simulink model "VSI_sw"  (R2019a)
settings: Solver=ode23t  StartTime=0  StopTime=0.2  MaxStep=2e-6  RelTol=1e-4  AbsTol=1e-5  EnableMultiTasking=on
values from neighbouring files (symbols this model uses):
  C = 22e-6    (= 2.2e-05)    [VSI_parameters_init.m]
  Ddref = 0.355    [VSI_parameters_init.m]
  Dqref = 0.11    [VSI_parameters_init.m]
  DT = 1e-6    (= 1e-06)    [VSI_parameters_init.m]
  fsw = 20e+3    (= 20000)    [VSI_parameters_init.m]
  Idref = 3*sqrt(3)    [VSI_parameters_init.m]
  Iqref = 0    [VSI_parameters_init.m]
  kii = 2*pi*fi*(RL)/Vdcref    (= 1.0471975512)    [VSI_parameters_init.m]
  kiv = 2*pi*fv/R    (= 41.8879020479)    [VSI_parameters_init.m]
  kpi = 2*pi*fi*L/Vdcref    (= 0.0251327412287)    [VSI_parameters_init.m]
  kpv = 2*pi*fv*C    (= 0.0138230076758)    [VSI_parameters_init.m]
  L = 1.2e-3    (= 0.0012)    [VSI_parameters_init.m]
  R = 15    [VSI_parameters_init.m]
  RL = 50e-3    (= 0.05)    [VSI_parameters_init.m]
  Vdc = 300    [VSI_parameters_init.m]
  Vdcref = 300    [VSI_parameters_init.m]
  Vdref = Vsdq(1)    [VSI_parameters_init.m]
  Vfd = 0.7    [VSI_parameters_init.m]
  Vfs = 1.2    [VSI_parameters_init.m]
  Vqref = Vsdq(2)    [VSI_parameters_init.m]
  w = 2*pi*f    (= 2513.27412287)    [VSI_parameters_init.m]
libraries: powerlib x20, simulink x2
settings Model: Creator=marko  LastModifiedBy=Dominion
settings SolverCC: AutoScaleAbsTol=off  MaxConsecutiveMinStep=10
settings DataIOCC: SaveFinalState=on  SaveFormat=Array  SignalLoggingSaveFormat=ModelDataLogs  ReturnWorkspaceOutputs=off
settings OptimizationCC: ExpressionDepthLimit=2147483647  LifeSpan=inf
settings DebuggingCC: UnderspecifiedInitializationDetection=Classic  MergeDetectMultiDrivingBlocksExec=none  SolverPrmCheckMsg=warning  FcnCallInpInsideContextMsg=warning  StateNameClashWarn=warning  SFUnexpectedBacktrackingDiag=warning  SFNoUnconditionalDefaultTransitionDiag=warning  SFExecutionAtInitializationDiag=none  ArithmeticOperatorsInVariantConditions=warning
settings HardwareCC: ProdBitPerPointer=32  ProdBitPerSizeT=32  ProdBitPerPtrDiffT=32  ProdLargestAtomicFloat=None  ProdIntDivRoundTo=Undefined  ProdEndianess=Unspecified  ProdWordSize=32  ProdHWDeviceType=32-bit Generic
settings ModelReferenceCC: PropagateSignalLabelsOutOfModel=off
settings SFSimCC: SimUseLocalCustomCode=off
settings RTWCC: RTWUseLocalCustomCode=off
settings CodeAppCC: StateflowObjectComments=on
settings GRTTargetCC: TargetLangStandard=C89/C90 (ANSI)  GeneratePreprocessorConditionals=Disable all  CombineOutputUpdateFcns=off  GRTInterface=on
settings ConfigComp: CovMetricSettings=dw  CovHtmlReporting=on  CovSaveCumulativeToWorkspaceVar=on  CovSaveSingleToWorkspaceVar=on  CovExternalEMLEnable=off

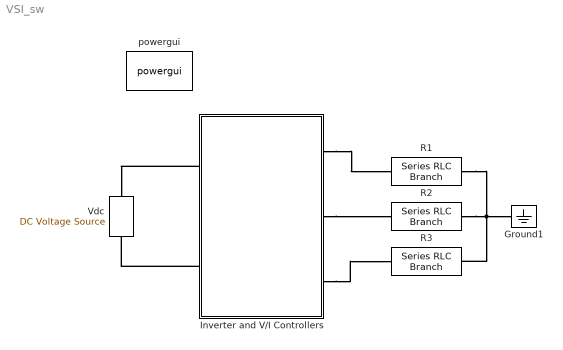
== system VSI_sw ==
  Ground1 : powerlib/Elements/Ground  LConnTagsString=a
      settings: SourceProductName=Simscape Electrical
  Inverter and V/I Controllers : Subsystem
  R1 : powerlib/Elements/Series RLC Branch  LConnTagsString=__new0  RConnTagsString=__new0  BranchType=RL  Resistance=R  Inductance=0.1*L  SetiL0=off  InitialCurrent=0  Capacitance=1e-6  Setx0=off  InitialVoltage=0  Measurements=None
      settings: SourceProductName=Simscape Electrical
  R2 : powerlib/Elements/Series RLC Branch  LConnTagsString=__new0  RConnTagsString=__new0  BranchType=RL  Resistance=R  Inductance=0.1*L  SetiL0=off  InitialCurrent=0  Capacitance=1e-6  Setx0=off  InitialVoltage=0  Measurements=None
      settings: SourceProductName=Simscape Electrical
  R3 : powerlib/Elements/Series RLC Branch  LConnTagsString=__new0  RConnTagsString=__new0  BranchType=RL  Resistance=R  Inductance=0.1*L  SetiL0=off  InitialCurrent=0  Capacitance=1e-6  Setx0=off  InitialVoltage=0  Measurements=None
      settings: SourceProductName=Simscape Electrical
  Vdc : powerlib/Electrical Sources/DC Voltage Source  Amplitude=Vdc  Measurements=None
      settings: SourceProductName=Simscape Electrical
  powergui : powerlib/powergui  Priority=1  SimulationMode=Continuous  SampleTime=50e-6  frequency=60  Iterations=50  frequencyindice=0  Pbase=100e6  ErrMax=1e-4  UnitsV=kV  UnitsW=MW  buscounter=0  FunctionMessages=off  echomessages=off  EnableUseOfTLC=off  CurrentSourceSwitches=off  DisableSnubberDevices=off  DisableRonSwitches=off  DisableVfSwitches=off  DisplayEquations=off  AutomaticDiscreteSolvers=off  SolverType=Tustin/Backward Euler (TBE)  Interpol=off  ExternalGateDelay=off  methode=off  Ts=0  x0status=blocks  SPID=on  SwTol=0  HookPort=off  NonlinearTolerance=0  nMaxIteration=15  ContinueOnMaxIteration=off  RestoreLinks=warning  ResistiveCurrentMeasurement=off  Frange=[0:2:500]  Ylog=off  Xlog=on  ShowGrid=off  save=off  variable=ZData  structure=0  ZoomFFT=on  StartTime=0.0  cycles=1  DisplayStyle=1  fundamental=60  FreqAxis=off  MaxFrequency=1000  frequencyindicesteady=400  RmsSteady=1  display=off
      settings: SourceProductName=Simscape Electrical
  connections:
  Inverter and V/I Controllers/LConn1 -- Vdc/RConn1
  Inverter and V/I Controllers/LConn2 -- Vdc/LConn1
  R1/RConn1 -- R3/RConn1 -- Ground1/LConn1 -- R2/RConn1
  Inverter and V/I Controllers/RConn1 -- R1/LConn1
  Inverter and V/I Controllers/RConn2 -- R2/LConn1
  Inverter and V/I Controllers/RConn3 -- R3/LConn1

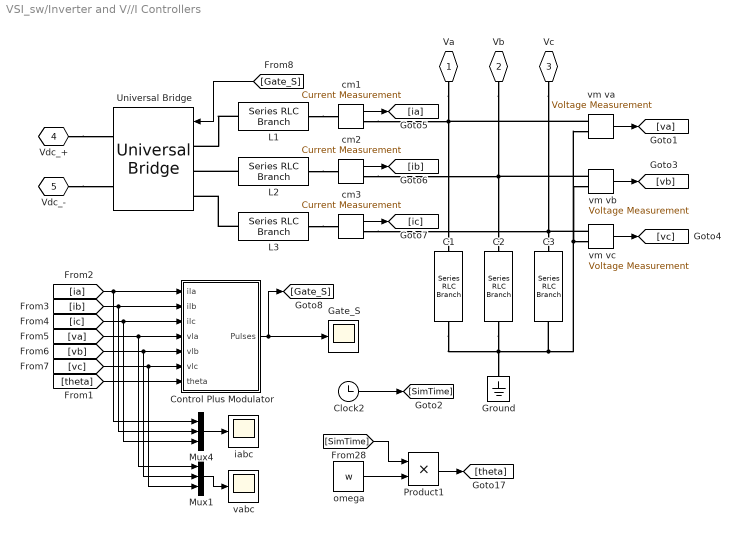
== system VSI_sw/Inverter and V//I Controllers ==
  C1 : powerlib/Elements/Series RLC Branch  LConnTagsString=__new0  RConnTagsString=__new0  BranchType=C  Resistance=1  Inductance=1e-3  SetiL0=off  InitialCurrent=0  Capacitance=C  Setx0=off  InitialVoltage=0  Measurements=None
      settings: SourceProductName=Simscape Electrical
  C2 : powerlib/Elements/Series RLC Branch  LConnTagsString=__new0  RConnTagsString=__new0  BranchType=C  Resistance=1  Inductance=1e-3  SetiL0=off  InitialCurrent=0  Capacitance=C  Setx0=off  InitialVoltage=0  Measurements=None
      settings: SourceProductName=Simscape Electrical
  C3 : powerlib/Elements/Series RLC Branch  LConnTagsString=__new0  RConnTagsString=__new0  BranchType=C  Resistance=1  Inductance=1e-3  SetiL0=off  InitialCurrent=0  Capacitance=C  Setx0=off  InitialVoltage=0  Measurements=None
      settings: SourceProductName=Simscape Electrical
  Clock2 : Clock
  Control Plus Modulator : Subsystem
  Gate_S : Scope
  Ground : powerlib/Elements/Ground  LConnTagsString=a
      settings: SourceProductName=Simscape Electrical
  L1 : powerlib/Elements/Series RLC Branch  LConnTagsString=__new0  RConnTagsString=__new0  BranchType=RL  Resistance=RL  Inductance=L  SetiL0=off  InitialCurrent=0  Capacitance=1e-6  Setx0=off  InitialVoltage=0  Measurements=None
      settings: SourceProductName=Simscape Electrical
  L2 : powerlib/Elements/Series RLC Branch  LConnTagsString=__new0  RConnTagsString=__new0  BranchType=RL  Resistance=RL  Inductance=L  SetiL0=off  InitialCurrent=0  Capacitance=1e-6  Setx0=off  InitialVoltage=0  Measurements=None
      settings: SourceProductName=Simscape Electrical
  L3 : powerlib/Elements/Series RLC Branch  LConnTagsString=__new0  RConnTagsString=__new0  BranchType=RL  Resistance=RL  Inductance=L  SetiL0=off  InitialCurrent=0  Capacitance=1e-6  Setx0=off  InitialVoltage=0  Measurements=None
      settings: SourceProductName=Simscape Electrical
  Mux1 : Mux  Inputs=3
  Mux4 : Mux  Inputs=3
  Product1 : Product  RndMeth=Zero
  Universal Bridge : powerlib/Power Electronics/Universal Bridge  Arms=3  SnubberResistance=inf  SnubberCapacitance=inf  Device=IGBT / Diodes  Ron=Rsd  Lon=0  ForwardVoltages=[Vfs Vfd]  ForwardVoltage=0  GTOparameters=[ 10e-6 , 20e-6 ]  IGBTparameters=[ 0, 0 ]  Measurements=None  Measurements_2=None  converterType=Rectifier
      settings: SourceProductName=Simscape Electrical
  cm1 : powerlib/Measurements/Current Measurement  PhasorSimulation=off  OutputType=Complex  PSBequivalent=0
      settings: SourceProductName=Simscape Electrical
  cm2 : powerlib/Measurements/Current Measurement  PhasorSimulation=off  OutputType=Complex  PSBequivalent=0
      settings: SourceProductName=Simscape Electrical
  cm3 : powerlib/Measurements/Current Measurement  PhasorSimulation=off  OutputType=Complex  PSBequivalent=0
      settings: SourceProductName=Simscape Electrical
  iabc : Scope
  omega : Constant  Value=w
  vabc : Scope
  vm va : powerlib/Measurements/Voltage Measurement  PhasorSimulation=off  OutputType=Complex  PSBequivalent=0
      settings: SourceProductName=Simscape Electrical
  vm vb : powerlib/Measurements/Voltage Measurement  PhasorSimulation=off  OutputType=Complex  PSBequivalent=0
      settings: SourceProductName=Simscape Electrical
  vm vc : powerlib/Measurements/Voltage Measurement  PhasorSimulation=off  OutputType=Complex  PSBequivalent=0
      settings: SourceProductName=Simscape Electrical
  Va : PMIOPort  Tag=PMCPort  Side=Right
  Vb : PMIOPort  Tag=PMCPort  Port=2  Side=Right
  Vc : PMIOPort  Tag=PMCPort  Port=3  Side=Right
  Vdc_+ : PMIOPort  Tag=PMCPort  Port=4  Side=Left
  Vdc_- : PMIOPort  Tag=PMCPort  Port=5  Side=Left
  wires:
  omega/1 -> Product1/2
  [SimTime] -> Product1/1
  Clock2/1 -> [SimTime]
  Product1/1 -> [theta]
  [theta] -> Control Plus Modulator/7(theta)
  Control Plus Modulator/1(Pulses) -> Gate_S/1, [Gate_S]
  Mux4/1 -> iabc/1
  vm va/1 -> [va]
  vm vb/1 -> [vb]
  vm vc/1 -> [vc]
  cm1/1 -> [ia]
  cm2/1 -> [ib]
  cm3/1 -> [ic]
  [ia] -> Control Plus Modulator/1(ila), Mux4/1
  [ib] -> Control Plus Modulator/2(ilb), Mux4/2
  [ic] -> Control Plus Modulator/3(ilc), Mux4/3
  [va] -> Control Plus Modulator/4(vla), Mux1/1
  [vb] -> Control Plus Modulator/5(vlb), Mux1/2
  [vc] -> Control Plus Modulator/6(vlc), Mux1/3
  Mux1/1 -> vabc/1
  [Gate_S] -> Universal Bridge/1
  connections:
  Va/RConn1 -- cm1/RConn1 -- C1/LConn1 -- vm va/LConn1
  C1/RConn1 -- C2/RConn1 -- Ground/LConn1 -- C3/RConn1 -- vm va/LConn2 -- vm vb/LConn2 -- vm vc/LConn2
  Vb/RConn1 -- cm2/RConn1 -- C2/LConn1 -- vm vb/LConn1
  Vc/RConn1 -- cm3/RConn1 -- C3/LConn1 -- vm vc/LConn1
  L1/LConn1 -- Universal Bridge/LConn1
  L1/RConn1 -- cm1/LConn1
  L2/LConn1 -- Universal Bridge/LConn2
  L2/RConn1 -- cm2/LConn1
  L3/LConn1 -- Universal Bridge/LConn3
  L3/RConn1 -- cm3/LConn1
  Vdc_+/RConn1 -- Universal Bridge/RConn1
  Vdc_-/RConn1 -- Universal Bridge/RConn2

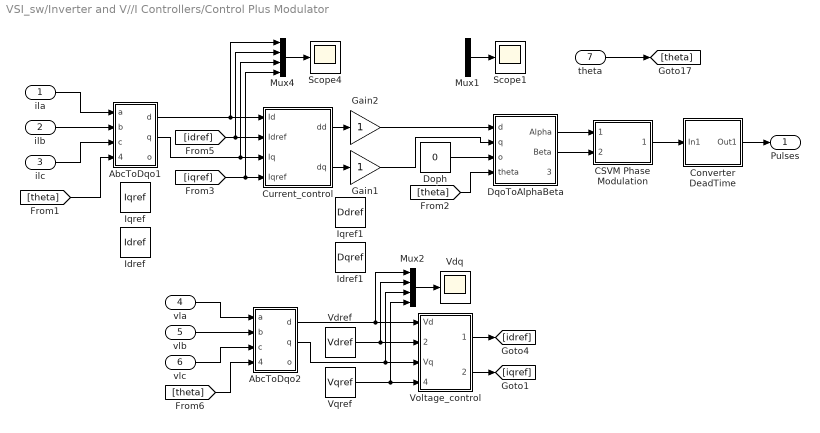
== system VSI_sw/Inverter and V//I Controllers/Control Plus Modulator ==
  ila : Inport
  ilb : Inport  Port=2
  ilc : Inport  Port=3
  vla : Inport  Port=4
  vlb : Inport  Port=5
  vlc : Inport  Port=6
  theta : Inport  Port=7
  AbcToDqo1 : Subsystem
  AbcToDqo2 : Subsystem
  CSVM Phase Modulation : Subsystem
  Converter DeadTime : Subsystem
  Current_control : Subsystem
  Doph : Constant  Value=0
  DqoToAlphaBeta : Subsystem
  Gain1 : Gain
  Gain2 : Gain
  Idref : Constant  Value=Idref
  Idref1 : Constant  Value=Dqref
  Iqref : Constant  Value=Iqref
  Iqref1 : Constant  Value=Ddref
  Mux1 : Mux  Inputs=2
  Mux2 : Mux
  Mux4 : Mux
  Scope1 : Scope
  Scope4 : Scope
  Vdq : Scope
  Vdref : Constant  Value=Vdref
  Voltage_control : Subsystem
  Vqref : Constant  Value=Vqref
  Pulses : Outport
  wires:
  AbcToDqo1/1(d) -> Current_control/1(Id), Mux4/1
  AbcToDqo1/2(q) -> Current_control/3(Iq), Mux4/3
  Current_control/1(dd) -> Gain2/1
  Current_control/2(dq) -> Gain1/1
  Mux4/1 -> Scope4/1
  ila/1 -> AbcToDqo1/1(a)
  ilb/1 -> AbcToDqo1/2(b)
  ilc/1 -> AbcToDqo1/3(c)
  theta/1 -> [theta]
  [theta] -> AbcToDqo1/4(theta)
  Mux1/1 -> Scope1/1
  DqoToAlphaBeta/1(Alpha) -> CSVM Phase Modulation/1(Dalpha)
  DqoToAlphaBeta/2(Beta) -> CSVM Phase Modulation/2(Dbeta)
  Doph/1 -> DqoToAlphaBeta/3(o)
  CSVM Phase Modulation/1(Pulses) -> Converter DeadTime/1(In1)
  [theta] -> DqoToAlphaBeta/4(theta)
  Converter DeadTime/1(Out1) -> Pulses/1
  Vqref/1 -> Voltage_control/4(Vqref), Mux2/4
  Vdref/1 -> Voltage_control/2(Vdref), Mux2/2
  AbcToDqo2/1(d) -> Voltage_control/1(Vd), Mux2/1
  AbcToDqo2/2(q) -> Voltage_control/3(Vq), Mux2/3
  Mux2/1 -> Vdq/1
  Voltage_control/1(idref) -> [idref]
  Voltage_control/2(iqref) -> [iqref]
  [idref] -> Current_control/2(Idref), Mux4/2
  [iqref] -> Current_control/4(Iqref), Mux4/4
  vla/1 -> AbcToDqo2/1(a)
  vlb/1 -> AbcToDqo2/2(b)
  vlc/1 -> AbcToDqo2/3(c)
  [theta] -> AbcToDqo2/4(theta)
  Gain2/1 -> DqoToAlphaBeta/1(d)
  Gain1/1 -> DqoToAlphaBeta/2(q)

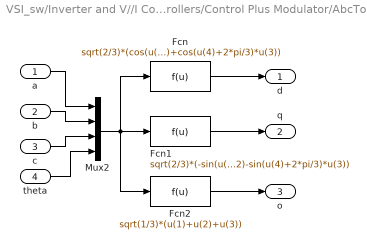
== system VSI_sw/Inverter and V//I Controllers/Control Plus Modulator/AbcToDqo1 ==
  a : Inport
  b : Inport  Port=2
  c : Inport  Port=3
  theta : Inport  Port=4
  Fcn : Fcn  Expr=sqrt(2/3)*(cos(u(4))*u(1)+cos(u(4)-2*pi/3)*u(2)+cos(u(4)+2*pi/3)*u(3))
  Fcn1 : Fcn  Expr=sqrt(2/3)*(-sin(u(4))*u(1)-sin(u(4)-2*pi/3)*u(2)-sin(u(4)+2*pi/3)*u(3))
  Fcn2 : Fcn  Expr=sqrt(1/3)*(u(1)+u(2)+u(3))
  Mux2 : Mux
  d : Outport
  q : Outport  Port=2
  o : Outport  Port=3
  wires:
  Fcn/1 -> d/1
  Fcn1/1 -> q/1
  a/1 -> Mux2/1
  b/1 -> Mux2/2
  c/1 -> Mux2/3
  theta/1 -> Mux2/4
  Mux2/1 -> Fcn/1, Fcn2/1, Fcn1/1
  Fcn2/1 -> o/1

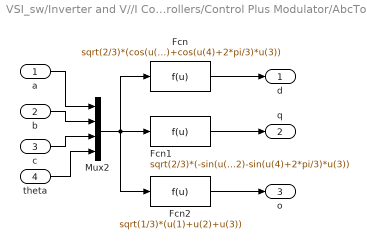
== system VSI_sw/Inverter and V//I Controllers/Control Plus Modulator/AbcToDqo2 ==
  a : Inport
  b : Inport  Port=2
  c : Inport  Port=3
  theta : Inport  Port=4
  Fcn : Fcn  Expr=sqrt(2/3)*(cos(u(4))*u(1)+cos(u(4)-2*pi/3)*u(2)+cos(u(4)+2*pi/3)*u(3))
  Fcn1 : Fcn  Expr=sqrt(2/3)*(-sin(u(4))*u(1)-sin(u(4)-2*pi/3)*u(2)-sin(u(4)+2*pi/3)*u(3))
  Fcn2 : Fcn  Expr=sqrt(1/3)*(u(1)+u(2)+u(3))
  Mux2 : Mux
  d : Outport
  q : Outport  Port=2
  o : Outport  Port=3
  wires:
  Fcn/1 -> d/1
  Fcn1/1 -> q/1
  a/1 -> Mux2/1
  b/1 -> Mux2/2
  c/1 -> Mux2/3
  theta/1 -> Mux2/4
  Mux2/1 -> Fcn/1, Fcn2/1, Fcn1/1
  Fcn2/1 -> o/1

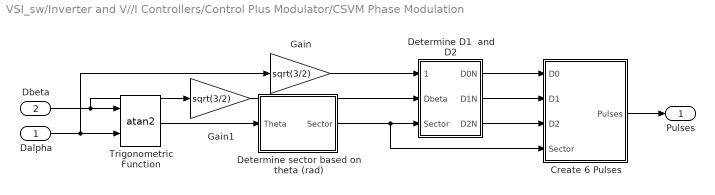
== system VSI_sw/Inverter and V//I Controllers/Control Plus Modulator/CSVM Phase Modulation ==
  Dalpha : Inport
  Dbeta : Inport  Port=2
  Create 6 Pulses : Subsystem
  Determine D1  and D2 : Subsystem
  Determine sector based on theta (rad) : Subsystem
  Gain : Gain  Gain=sqrt(3/2)
  Gain1 : Gain  Gain=sqrt(3/2)
  Trigonometric Function : Trigonometry  Operator=atan2
  Pulses : Outport
  wires:
  Dbeta/1 -> Trigonometric Function/1, Gain1/1
  Dalpha/1 -> Trigonometric Function/2, Gain/1
  Trigonometric Function/1 -> Determine sector based on theta (rad)/1(Theta)
  Determine sector based on theta (rad)/1(Sector) -> Determine D1  and D2/3(Sector), Create 6 Pulses/4(Sector)
  Gain/1 -> Determine D1  and D2/1(Dalpha)
  Gain1/1 -> Determine D1  and D2/2(Dbeta)
  Determine D1  and D2/1(D0N) -> Create 6 Pulses/1(D0)
  Create 6 Pulses/1(Pulses) -> Pulses/1
  Determine D1  and D2/2(D1N) -> Create 6 Pulses/2(D1)
  Determine D1  and D2/3(D2N) -> Create 6 Pulses/3(D2)

== system VSI_sw/Inverter and V//I Controllers/Control Plus Modulator/Converter DeadTime ==
  In1 : Inport
  Compare To Zero : simulink/Logic and Bit Operations/Compare To Zero  relop=<=  OutDataTypeStr=boolean
  Switch : Switch  Criteria=u2 ~= 0
  Transport Delay : TransportDelay  DelayTime=DT
  Out1 : Outport
  wires:
  In1/1 -> Switch/1, Compare To Zero/1, Transport Delay/1
  Transport Delay/1 -> Switch/3
  Compare To Zero/1 -> Switch/2
  Switch/1 -> Out1/1

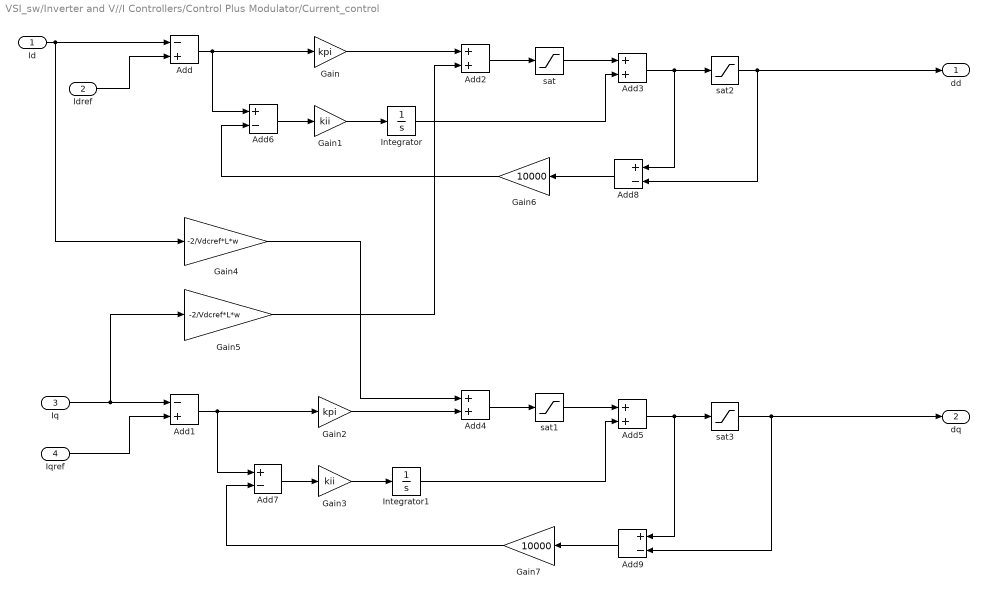
== system VSI_sw/Inverter and V//I Controllers/Control Plus Modulator/Current_control ==
  Id : Inport
  Idref : Inport  Port=2
  Iq : Inport  Port=3
  Iqref : Inport  Port=4
  Add : Sum  Inputs=-+
  Add1 : Sum  Inputs=-+
  Add{2..5} (4 alike) : Sum
  Add{6..9} (4 alike) : Sum  Inputs=+-
  Gain : Gain  Gain=kpi
  Gain1 : Gain  Gain=kii
  Gain2 : Gain  Gain=kpi
  Gain3 : Gain  Gain=kii
  Gain4 : Gain  Gain=-2/Vdcref*L*w
  Gain5 : Gain  Gain=-2/Vdcref*L*w
  Gain6 : Gain  Gain=10000
  Gain7 : Gain  Gain=10000
  Integrator : Integrator
  Integrator1 : Integrator
  sat{,1..3} (4 alike) : Saturate  UpperLimit=1  LowerLimit=-1
  dd : Outport
  dq : Outport  Port=2
  wires:
  Id/1 -> Gain4/1, Add/1
  Idref/1 -> Add/2
  Iq/1 -> Gain5/1, Add1/1
  Iqref/1 -> Add1/2
  Add/1 -> Gain/1, Add6/1
  Gain1/1 -> Integrator/1
  Add2/1 -> sat/1
  sat/1 -> Add3/1
  Integrator/1 -> Add3/2
  Gain/1 -> Add2/1
  Add1/1 -> Gain2/1, Add7/1
  Gain3/1 -> Integrator1/1
  Gain2/1 -> Add4/2
  Add4/1 -> sat1/1
  sat1/1 -> Add5/1
  Integrator1/1 -> Add5/2
  sat2/1 -> Add8/2, dd/1
  Add5/1 -> sat3/1, Add9/1
  sat3/1 -> Add9/2, dq/1
  Add6/1 -> Gain1/1
  Add7/1 -> Gain3/1
  Add3/1 -> Add8/1, sat2/1
  Add8/1 -> Gain6/1
  Add9/1 -> Gain7/1
  Gain6/1 -> Add6/2
  Gain7/1 -> Add7/2
  Gain4/1 -> Add4/1
  Gain5/1 -> Add2/2

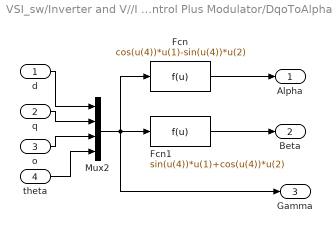
== system VSI_sw/Inverter and V//I Controllers/Control Plus Modulator/DqoToAlphaBeta ==
  d : Inport
  q : Inport  Port=2
  o : Inport  Port=3
  theta : Inport  Port=4
  Fcn : Fcn  Expr=cos(u(4))*u(1)-sin(u(4))*u(2)
  Fcn1 : Fcn  Expr=sin(u(4))*u(1)+cos(u(4))*u(2)
  Mux2 : Mux
  Alpha : Outport
  Beta : Outport  Port=2
  Gamma : Outport  Port=3
  wires:
  d/1 -> Mux2/1
  q/1 -> Mux2/2
  o/1 -> Mux2/3
  theta/1 -> Mux2/4
  Mux2/1 -> Fcn/1, Fcn1/1, Gamma/1
  Fcn1/1 -> Beta/1
  Fcn/1 -> Alpha/1

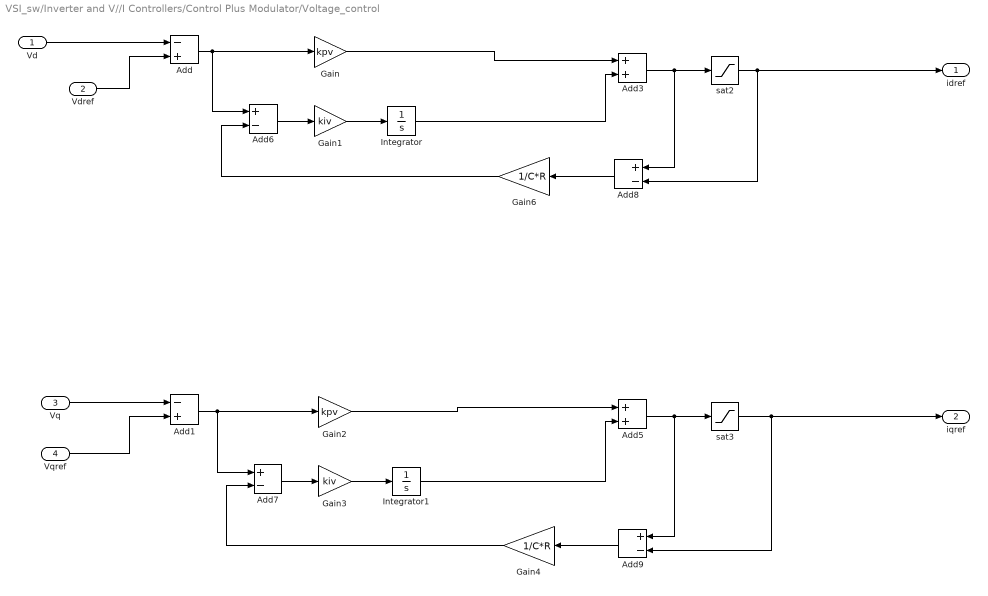
== system VSI_sw/Inverter and V//I Controllers/Control Plus Modulator/Voltage_control ==
  Vd : Inport
  Vdref : Inport  Port=2
  Vq : Inport  Port=3
  Vqref : Inport  Port=4
  Add : Sum  Inputs=-+
  Add1 : Sum  Inputs=-+
  Add3 : Sum
  Add5 : Sum
  Add{6..9} (4 alike) : Sum  Inputs=+-
  Gain : Gain  Gain=kpv
  Gain1 : Gain  Gain=kiv
  Gain2 : Gain  Gain=kpv
  Gain3 : Gain  Gain=kiv
  Gain4 : Gain  Gain=1/C*R
  Gain6 : Gain  Gain=1/C*R
  Integrator : Integrator
  Integrator1 : Integrator
  sat2 : Saturate  UpperLimit=40  LowerLimit=-40
  sat3 : Saturate  UpperLimit=40  LowerLimit=-40
  idref : Outport
  iqref : Outport  Port=2
  wires:
  Gain4/1 -> Add7/2
  Gain6/1 -> Add6/2
  Add9/1 -> Gain4/1
  Add8/1 -> Gain6/1
  Add3/1 -> sat2/1, Add8/1
  Add7/1 -> Gain3/1
  Add6/1 -> Gain1/1
  sat3/1 -> iqref/1, Add9/2
  Add5/1 -> Add9/1, sat3/1
  sat2/1 -> idref/1, Add8/2
  Integrator1/1 -> Add5/2
  Gain2/1 -> Add5/1
  Gain3/1 -> Integrator1/1
  Add1/1 -> Add7/1, Gain2/1
  Gain/1 -> Add3/1
  Integrator/1 -> Add3/2
  Gain1/1 -> Integrator/1
  Add/1 -> Add6/1, Gain/1
  Vqref/1 -> Add1/2
  Vq/1 -> Add1/1
  Vdref/1 -> Add/2
  Vd/1 -> Add/1

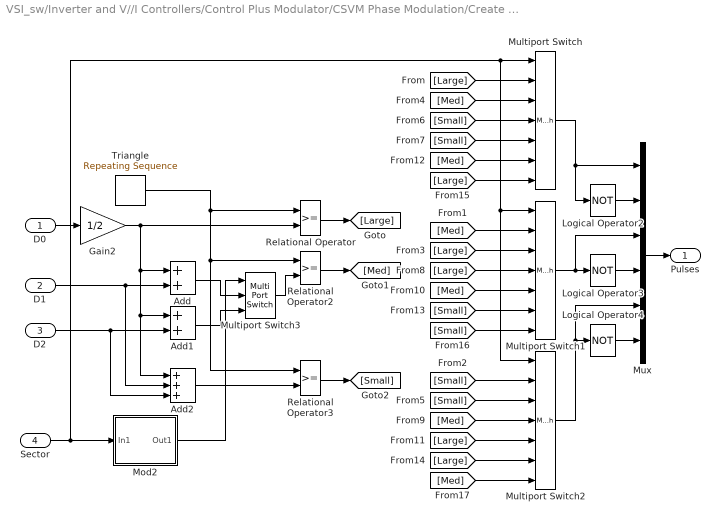
== system VSI_sw/Inverter and V//I Controllers/Control Plus Modulator/CSVM Phase Modulation/Create 6 Pulses ==
  D0 : Inport
  D1 : Inport  Port=2
  D2 : Inport  Port=3
  Sector : Inport  Port=4
  Add : Sum
  Add1 : Sum
  Add2 : Sum  Inputs=+++
  Gain2 : Gain  Gain=1/2
  Logical Operator2 : Logic  Operator=NOT  OutDataTypeStr=float('double')
  Logical Operator3 : Logic  Operator=NOT  OutDataTypeStr=float('double')
  Logical Operator4 : Logic  Operator=NOT  OutDataTypeStr=float('double')
  Mod2 : Subsystem
  Multiport Switch : MultiPortSwitch  Inputs=6  SaturateOnIntegerOverflow=on  InputSameDT=on
  Multiport Switch1 : MultiPortSwitch  Inputs=6  SaturateOnIntegerOverflow=on  InputSameDT=on
  Multiport Switch2 : MultiPortSwitch  Inputs=6  SaturateOnIntegerOverflow=on  InputSameDT=on
  Multiport Switch3 : MultiPortSwitch  Inputs=2
  Mux : Mux  Inputs=6
  Relational Operator : RelationalOperator  OutDataTypeStr=float('double')  RndMeth=Nearest  InputSameDT=on
  Relational Operator2 : RelationalOperator  OutDataTypeStr=float('double')  RndMeth=Nearest  InputSameDT=on
  Relational Operator3 : RelationalOperator  OutDataTypeStr=float('double')  RndMeth=Nearest  InputSameDT=on
  Triangle : simulink/Sources/Repeating Sequence  rep_seq_t=[0 0.5/fsw 1/fsw]  rep_seq_y=[0 1 0]
  Pulses : Outport
  wires:
  [Med] -> Multiport Switch2/7
  [Small] -> Multiport Switch1/7
  [Large] -> Multiport Switch/7
  [Large] -> Multiport Switch2/6
  [Small] -> Multiport Switch1/6
  [Med] -> Multiport Switch/6
  [Large] -> Multiport Switch2/5
  [Med] -> Multiport Switch1/5
  [Med] -> Multiport Switch2/4
  [Large] -> Multiport Switch1/4
  [Small] -> Multiport Switch/5
  [Small] -> Multiport Switch/4
  [Small] -> Multiport Switch2/3
  [Med] -> Multiport Switch/3
  [Large] -> Multiport Switch1/3
  [Small] -> Multiport Switch2/2
  [Med] -> Multiport Switch1/2
  [Large] -> Multiport Switch/2
  Multiport Switch3/1 -> Relational Operator2/2
  Relational Operator3/1 -> [Small]
  Relational Operator2/1 -> [Med]
  Relational Operator/1 -> [Large]
  Mod2/1(Out1) -> Multiport Switch3/1
  Add1/1 -> Multiport Switch3/3
  Add/1 -> Multiport Switch3/2
  Add2/1 -> Relational Operator3/2
  D2/1 -> Add2/3, Add1/2
  D1/1 -> Add2/2, Add/2
  Gain2/1 -> Relational Operator/2, Add/1, Add1/1, Add2/1
  Multiport Switch2/1 -> Logical Operator4/1, Mux/5
  Multiport Switch1/1 -> Logical Operator3/1, Mux/3
  Multiport Switch/1 -> Logical Operator2/1, Mux/1
  Logical Operator4/1 -> Mux/6
  Logical Operator3/1 -> Mux/4
  Logical Operator2/1 -> Mux/2
  Triangle/1 -> Relational Operator/1, Relational Operator2/1, Relational Operator3/1
  Sector/1 -> Mod2/1(In1), Multiport Switch/1, Multiport Switch1/1, Multiport Switch2/1
  D0/1 -> Gain2/1
  Mux/1 -> Pulses/1

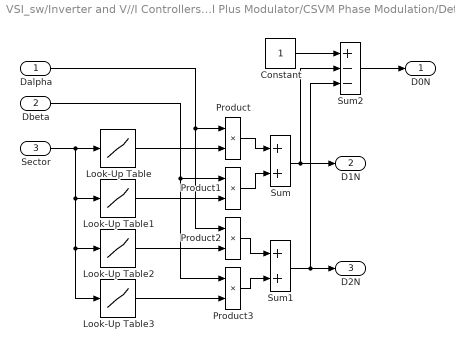
== system VSI_sw/Inverter and V//I Controllers/Control Plus Modulator/CSVM Phase Modulation/Determine D1  and D2 ==
  Dalpha : Inport
  Dbeta : Inport  Port=2
  Sector : Inport  Port=3
  Constant : Constant
  Look-Up Table : Lookup  InputValues=[1 2 3 4 5 6]  Table=[1 1 0 -1 -1 0]  SaturateOnIntegerOverflow=on
  Look-Up Table1 : Lookup  InputValues=[1 2 3 4 5 6]  Table=[-1/sqrt(3) 1/sqrt(3) 2/sqrt(3) 1/sqrt(3) -1/sqrt(3) -2/sqrt(3)]  SaturateOnIntegerOverflow=on
  Look-Up Table2 : Lookup  InputValues=[1 2 3 4 5 6]  Table=[0 -1 -1 0 1 1]  SaturateOnIntegerOverflow=on
  Look-Up Table3 : Lookup  InputValues=[1 2 3 4 5 6]  Table=[2/sqrt(3) 1/sqrt(3) -1/sqrt(3) -2/sqrt(3) -1/sqrt(3) 1/sqrt(3)]  SaturateOnIntegerOverflow=on
  Product{,1..3} (4 alike) : Product  SaturateOnIntegerOverflow=on  InputSameDT=on  OutDataTypeStr=Inherit: Same as first input
  Sum : Sum  SaturateOnIntegerOverflow=on  InputSameDT=on  OutDataTypeStr=Inherit: Same as first input
  Sum1 : Sum  SaturateOnIntegerOverflow=on  InputSameDT=on  OutDataTypeStr=Inherit: Same as first input
  Sum2 : Sum  Inputs=+--  SaturateOnIntegerOverflow=on  InputSameDT=on  OutDataTypeStr=Inherit: Same as first input
  D0N : Outport
  D1N : Outport  Port=2
  D2N : Outport  Port=3
  wires:
  Sum1/1 -> D2N/1, Sum2/3
  Sum/1 -> D1N/1, Sum2/2
  Product3/1 -> Sum1/2
  Product2/1 -> Sum1/1
  Product1/1 -> Sum/2
  Product/1 -> Sum/1
  Look-Up Table3/1 -> Product3/2
  Look-Up Table2/1 -> Product2/2
  Look-Up Table1/1 -> Product1/2
  Dbeta/1 -> Product3/1, Product1/1
  Look-Up Table/1 -> Product/2
  Dalpha/1 -> Product2/1, Product/1
  Sector/1 -> Look-Up Table3/1, Look-Up Table2/1, Look-Up Table1/1, Look-Up Table/1
  Constant/1 -> Sum2/1
  Sum2/1 -> D0N/1

== system VSI_sw/Inverter and V//I Controllers/Control Plus Modulator/CSVM Phase Modulation/Determine sector based on theta (rad) ==
  Theta : Inport
  Add : Sum  Inputs=+-
  Fcn2 : Fcn  Expr=(u(1)-1)/2
  Gain1 : Gain  Gain=2*pi
  "Look-Up Table Determine the sector of U* based on theta (rad). " : Lookup  InputValues=[0 pi/3 2*pi/3 pi 4*pi/3 5*pi/3 2*pi ]  Table=[1 2 3 4 5 6 6.5]  SaturateOnIntegerOverflow=on
  Rounding Function : Rounding
  Sign : Signum
  Sector : Outport
  wires:
  "Look-Up Table Determine the sector of U* based on theta (rad). "/1 -> Rounding Function/1
  Rounding Function/1 -> Sector/1
  Theta/1 -> Add/1, Sign/1
  Add/1 -> "Look-Up Table Determine the sector of U* based on theta (rad). "/1
  Gain1/1 -> Add/2
  Sign/1 -> Fcn2/1
  Fcn2/1 -> Gain1/1

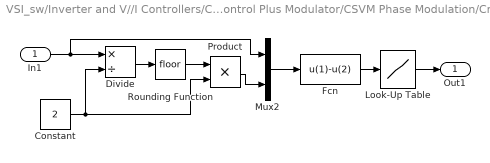
== system VSI_sw/Inverter and V//I Controllers/Control Plus Modulator/CSVM Phase Modulation/Create 6 Pulses/Mod2 ==
  In1 : Inport
  Constant : Constant  Value=2
  Divide : Product  Inputs=*/
  Fcn : Fcn  Expr=u(1)-u(2)
  Look-Up Table : Lookup  InputValues=[0 1]  Table=[2 1]  SaturateOnIntegerOverflow=on
  Mux2 : Mux  Inputs=2
  Product : Product  RndMeth=Zero
  Rounding Function : Rounding
  Out1 : Outport
  wires:
  Constant/1 -> Divide/2, Product/2
  Divide/1 -> Rounding Function/1
  Rounding Function/1 -> Product/1
  Mux2/1 -> Fcn/1
  Product/1 -> Mux2/2
  Fcn/1 -> Look-Up Table/1
  In1/1 -> Divide/1, Mux2/1
  Look-Up Table/1 -> Out1/1
